simulink model "SAR_AOCS_Model"  (R2024a)
settings: Solver=VariableStepAuto  StartTime=0.0  StopTime=1000  RelTol=1e-3
values from neighbouring files (symbols this model uses):
  Q = 1e-10    [init_SAR_AOCS.m]
  Rgyro = 1e-12    [init_SAR_AOCS.m]
  Rstr = 1e-12    [init_SAR_AOCS.m]
  Ts = sim.dt    [init_SAR_AOCS.m]
  unit7 = ones(7,1)    [init_SAR_AOCS.m]
undefined symbols (not defined in the file or in its folder): initial, sim
libraries: simulink x3, slpidlib x3, sharedtransform x3, sharedTrackingLibrary x1, simulink_extras x1
settings Model: SimulationMode=accelerator  Creator=hendr  LastModifiedBy=hendr

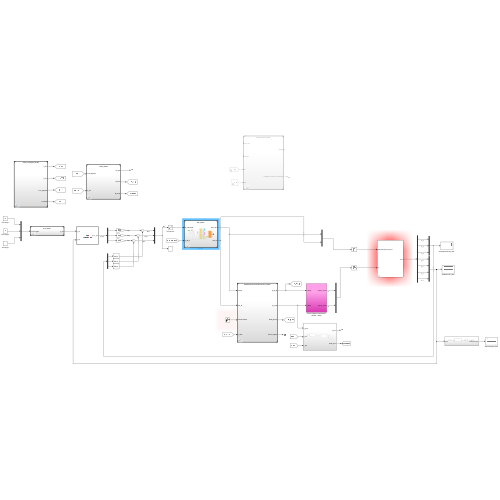
[thumbnail: Simulink's stored preview of the top-level diagram]
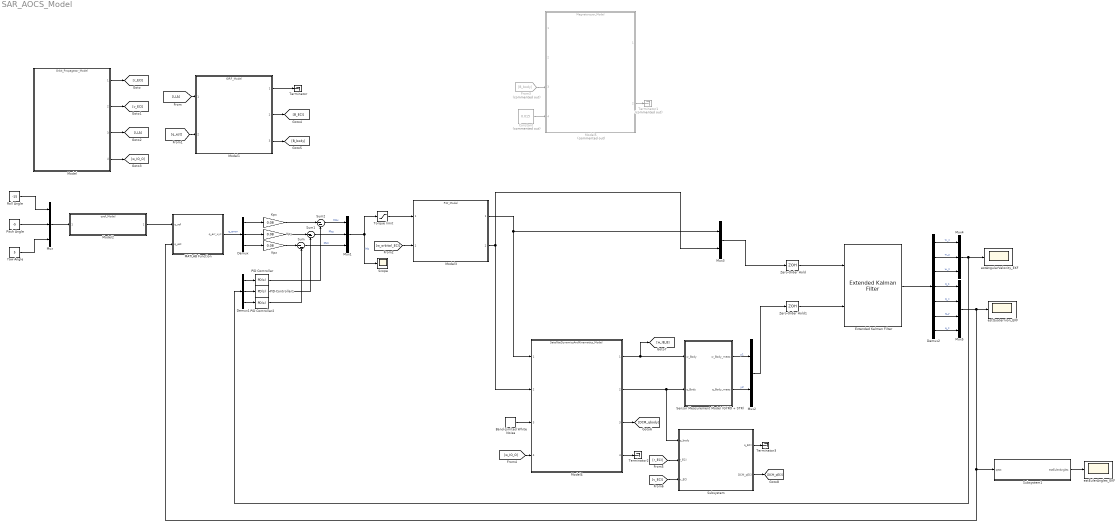
== system SAR_AOCS_Model ==
  Band-Limited White Noise : simulink/Sources/Band-Limited White Noise  Cov=Q*sim.dt  Ts=sim.dt  seed=[23341]
  Constant : Constant  Commented=on  Value=0.015
  Demux : Demux  Outputs=3
  Demux1 : Demux  Outputs=3
  Demux2 : Demux  Outputs=7
  Extended Kalman Filter : sharedTrackingLibrary/Extended Kalman Filter  StateTransitionFcn=dynamicFunctions2  HasStateTransitionJacobianFcn=off  HasAdditiveProcessNoise=Additive  ProcessNoise=diag(unit7)*Q  HasTimeVaryingProcessNoise=off  HasStateTransitionFcnExtraArgument=1  InitialState=[initial.omega, initial.q]  InitialStateCovariance=1e-6  MeasurementFcn1=measurementFunction2  HasMeasurementJacobianFcn1=off  HasMeasurementEnablePort1=off  HasAdditiveMeasurementNoise1=Additive  MeasurementNoise1=Rconf4  HasTimeVaryingMeasurementNoise1=off  HasMeasurementFcnExtraArgument1=0  HasMeasurementWrapping1=off  MeasurementFcn2=myMeasurementFcn  HasMeasurementJacobianFcn2=off  HasMeasurementEnablePort2=off  HasAdditiveMeasurementNoise2=Additive  MeasurementNoise2=1  HasTimeVaryingMeasurementNoise2=off  HasMeasurementFcnExtraArgument2=0  HasMeasurementWrapping2=off  MeasurementFcn3=myMeasurementFcn  HasMeasurementJacobianFcn3=off  HasMeasurementEnablePort3=off  HasAdditiveMeasurementNoise3=Additive  MeasurementNoise3=1  HasTimeVaryingMeasurementNoise3=off  HasMeasurementFcnExtraArgument3=0  HasMeasurementWrapping3=off  MeasurementFcn4=myMeasurementFcn  HasMeasurementJacobianFcn4=off  HasMeasurementEnablePort4=off  HasAdditiveMeasurementNoise4=Additive  MeasurementNoise4=1  HasTimeVaryingMeasurementNoise4=off  HasMeasurementFcnExtraArgument4=0  HasMeasurementWrapping4=off  MeasurementFcn5=myMeasurementFcn  HasMeasurementJacobianFcn5=off  HasMeasurementEnablePort5=off  HasAdditiveMeasurementNoise5=Additive  MeasurementNoise5=1  HasTimeVaryingMeasurementNoise5=off  HasMeasurementFcnExtraArgument5=0  HasMeasurementWrapping5=off  EnableMultirate=off  StateTransitionFcnSampleTime=1  MeasurementFcn1SampleTime=1  MeasurementFcn2SampleTime=1  MeasurementFcn3SampleTime=1  MeasurementFcn4SampleTime=1  MeasurementFcn5SampleTime=1  UseCurrentEstimator=on  OutputStateCovariance=off  DataType=double  SampleTime=Ts  NumberOfMeasurements=1
  From3 : From  Commented=on  GotoTag=B_body
  Kpx : Gain  Gain=0.08
  Kpy : Gain  Gain=0.08
  Kpz : Gain  Gain=0.08
  MATLAB Function : MATLAB Function  TreatAsAtomicUnit=on
  Model : ModelReference  ModelNameDialog=Orbit_Propagator_Model.slx  SimulationMode=Normal  ModelReferenceVersion=1.1
  Model1 : ModelReference  ModelNameDialog=IGRF_Model.slx  SimulationMode=Normal  ModelReferenceVersion=1.3
  Model2 : ModelReference  ModelNameDialog=qref_Model.slx  SimulationMode=Normal  ModelReferenceVersion=1.2
  Model3 : ModelReference  ModelNameDialog=RW_Model.slx  SimulationMode=Normal  ModelReferenceVersion=1.2
  Model4 : ModelReference  ModelNameDialog=SatelliteDynamicsAndKinematics_Model.slx  SimulationMode=Normal  ModelReferenceVersion=1.1
  Model5 : ModelReference  Commented=on  ModelNameDialog=Magnetorquer_Model.slx  SimulationMode=Normal  ModelReferenceVersion=1.3
  Mux : Mux  Inputs=3
  Mux1 : Mux  Inputs=3
  Mux2 : Mux  Inputs=2
  Mux3 : Mux  Inputs=2
  Mux4 : Mux  Inputs=3
  Mux5 : Mux
  PID Controller : slpidlib/PID Controller  Controller=PD  Form=Parallel  TimeDomain=Continuous-time  UseExternalTs=off  SampleTime=-1  IntegratorMethod=Forward Euler  FilterMethod=Forward Euler  ControllerParametersSource=internal  P=1  I=1  UseKiTs=off  D=2  UseExternalDerivativeSource=off  N=100  UseFilter=on  TunerSelectOption=Transfer Function Based (PID Tuner App)  InitialConditionSource=internal  InitialConditionForIntegrator=0  InitialConditionForFilter=0  DifferentiatorICPrevScaledInput=0  ExternalReset=none  TrackingMode=off  Kt=1  LimitOutput=off  SatLimitsSource=internal  UpperSaturationLimit=inf  LowerSaturationLimit=-inf  LinearizeAsGain=on  AntiWindupMode=none  Kb=1  LimitIntegrator=off  UpperIntegratorSaturationLimit=inf  LowerIntegratorSaturationLimit=-inf  POutMin=[]  POutMax=[]  IOutMin=[]  IOutMax=[]  DOutMin=[]  DOutMax=[]  NOutMin=[]  NOutMax=[]  SumOutMin=[]  SumOutMax=[]  SaturationOutMin=[]  SaturationOutMax=[]  PParamMin=[]  PParamMax=[]  IParamMin=[]  IParamMax=[]  DParamMin=[]  DParamMax=[]  NParamMin=[]  NParamMax=[]  KbParamMin=[]  KbParamMax=[]  KtParamMin=[]  KtParamMax=[]  KbOutMin=[]  KbOutMax=[]  KtOutMin=[]  KtOutMax=[]  IntegratorOutMin=[]  IntegratorOutMax=[]  FilterOutMin=[]  FilterOutMax=[]  SumI1OutMin=[]  SumI1OutMax=[]  SumI2OutMin=[]  SumI2OutMax=[]  SumI3OutMin=[]  SumI3OutMax=[]  SumI4OutMin=[]  SumI4OutMax=[]  SumDOutMin=[]  SumDOutMax=[]  DifferentiatorOutMin=[]  DifferentiatorOutMax=[]  FilterDiffOutCoefMin=[]  FilterDiffOutCoefMax=[]  ReciprocalOutMin=[]  ReciprocalOutMax=[]  SumDenOutMin=[]  SumDenOutMax=[]  SumNumOutMin=[]  SumNumOutMax=[]  DivideOutMin=[]  DivideOutMax=[]  UdiffTsProdOutMin=[]  UdiffTsProdOutMax=[]  NTsProdOutMin=[]  NTsProdOutMax=[]  UintegralTsProdOutMin=[]  UintegralTsProdOutMax=[]  UngainTsProdOutMin=[]  UngainTsProdOutMax=[]  ClampingZeroOutDataTypeStr=Inherit: Inherit via back propagation  ClampingZeroOutMin=[]  ClampingZeroOutMax=[]  FilterDenConstantOutDataTypeStr=Inherit: Inherit via back propagation  FilterDenConstantOutMin=[]  FilterDenConstantOutMax=[]  PCopyOutDataTypeStr=Inherit: Inherit via back propagation  PCopyOutMin=[]  PCopyOutMax=[]  NCopyOutDataTypeStr=Inherit: Inherit via back propagation  NCopyOutMin=[]  NCopyOutMax=[]  IntegratorContinuousStateAttributes=''  IntegratorStateMustResolveToSignalObject=off  IntegratorRTWStateStorageClass=Auto  FilterContinuousStateAttributes=''  FilterStateMustResolveToSignalObject=off  FilterRTWStateStorageClass=Auto  ParallelPVariant=InternalParameters  IdealPVariant=Disabled  IVariant=Disabled  DVariant=InternalParameters  IntegratorVariant=Disabled  SatVariant=Disabled  AWVariant=Disabled  PCopyVariant=Disabled  TRVariant=Disabled  FdbkBlocksVariant=Forward  IdealPFdbkVariant=Disabled  SatFdbkVariant=Disabled  DerivativeFilterVariant=ContFilter  NVariant=InternalParameters  NCopyVariant=Disabled  FilterICVariant=InternalICsFilter  IntegratorICVariant=Disabled  ExternalResetVariant=Disabled  TRSumVariant=Passthrough  SumFdbkVariant=Disabled  SumVariant=Sum_PD  TsampFilterVariant=InternalTs  TsampNgainVariant=Passthrough  TsampIntegralVariant=Disabled_SignalSpec  ExternalSaturationOutDataTypeStr=Inherit: Same as second input  DerivativeSourceVariant=ErrorSignal
  PID Controller1 : slpidlib/PID Controller  Controller=PD  Form=Parallel  TimeDomain=Continuous-time  UseExternalTs=off  SampleTime=-1  IntegratorMethod=Forward Euler  FilterMethod=Forward Euler  ControllerParametersSource=internal  P=1  I=1  UseKiTs=off  D=2  UseExternalDerivativeSource=off  N=100  UseFilter=on  TunerSelectOption=Transfer Function Based (PID Tuner App)  InitialConditionSource=internal  InitialConditionForIntegrator=0  InitialConditionForFilter=0  DifferentiatorICPrevScaledInput=0  ExternalReset=none  TrackingMode=off  Kt=1  LimitOutput=off  SatLimitsSource=internal  UpperSaturationLimit=inf  LowerSaturationLimit=-inf  LinearizeAsGain=on  AntiWindupMode=none  Kb=1  LimitIntegrator=off  UpperIntegratorSaturationLimit=inf  LowerIntegratorSaturationLimit=-inf  POutMin=[]  POutMax=[]  IOutMin=[]  IOutMax=[]  DOutMin=[]  DOutMax=[]  NOutMin=[]  NOutMax=[]  SumOutMin=[]  SumOutMax=[]  SaturationOutMin=[]  SaturationOutMax=[]  PParamMin=[]  PParamMax=[]  IParamMin=[]  IParamMax=[]  DParamMin=[]  DParamMax=[]  NParamMin=[]  NParamMax=[]  KbParamMin=[]  KbParamMax=[]  KtParamMin=[]  KtParamMax=[]  KbOutMin=[]  KbOutMax=[]  KtOutMin=[]  KtOutMax=[]  IntegratorOutMin=[]  IntegratorOutMax=[]  FilterOutMin=[]  FilterOutMax=[]  SumI1OutMin=[]  SumI1OutMax=[]  SumI2OutMin=[]  SumI2OutMax=[]  SumI3OutMin=[]  SumI3OutMax=[]  SumI4OutMin=[]  SumI4OutMax=[]  SumDOutMin=[]  SumDOutMax=[]  DifferentiatorOutMin=[]  DifferentiatorOutMax=[]  FilterDiffOutCoefMin=[]  FilterDiffOutCoefMax=[]  ReciprocalOutMin=[]  ReciprocalOutMax=[]  SumDenOutMin=[]  SumDenOutMax=[]  SumNumOutMin=[]  SumNumOutMax=[]  DivideOutMin=[]  DivideOutMax=[]  UdiffTsProdOutMin=[]  UdiffTsProdOutMax=[]  NTsProdOutMin=[]  NTsProdOutMax=[]  UintegralTsProdOutMin=[]  UintegralTsProdOutMax=[]  UngainTsProdOutMin=[]  UngainTsProdOutMax=[]  ClampingZeroOutDataTypeStr=Inherit: Inherit via back propagation  ClampingZeroOutMin=[]  ClampingZeroOutMax=[]  FilterDenConstantOutDataTypeStr=Inherit: Inherit via back propagation  FilterDenConstantOutMin=[]  FilterDenConstantOutMax=[]  PCopyOutDataTypeStr=Inherit: Inherit via back propagation  PCopyOutMin=[]  PCopyOutMax=[]  NCopyOutDataTypeStr=Inherit: Inherit via back propagation  NCopyOutMin=[]  NCopyOutMax=[]  IntegratorContinuousStateAttributes=''  IntegratorStateMustResolveToSignalObject=off  IntegratorRTWStateStorageClass=Auto  FilterContinuousStateAttributes=''  FilterStateMustResolveToSignalObject=off  FilterRTWStateStorageClass=Auto  ParallelPVariant=InternalParameters  IdealPVariant=Disabled  IVariant=Disabled  DVariant=InternalParameters  IntegratorVariant=Disabled  SatVariant=Disabled  AWVariant=Disabled  PCopyVariant=Disabled  TRVariant=Disabled  FdbkBlocksVariant=Forward  IdealPFdbkVariant=Disabled  SatFdbkVariant=Disabled  DerivativeFilterVariant=ContFilter  NVariant=InternalParameters  NCopyVariant=Disabled  FilterICVariant=InternalICsFilter  IntegratorICVariant=Disabled  ExternalResetVariant=Disabled  TRSumVariant=Passthrough  SumFdbkVariant=Disabled  SumVariant=Sum_PD  TsampFilterVariant=InternalTs  TsampNgainVariant=Passthrough  TsampIntegralVariant=Disabled_SignalSpec  ExternalSaturationOutDataTypeStr=Inherit: Same as second input  DerivativeSourceVariant=ErrorSignal
  PID Controller2 : slpidlib/PID Controller  Controller=PD  Form=Parallel  TimeDomain=Continuous-time  UseExternalTs=off  SampleTime=-1  IntegratorMethod=Forward Euler  FilterMethod=Forward Euler  ControllerParametersSource=internal  P=1  I=1  UseKiTs=off  D=2  UseExternalDerivativeSource=off  N=100  UseFilter=on  TunerSelectOption=Transfer Function Based (PID Tuner App)  InitialConditionSource=internal  InitialConditionForIntegrator=0  InitialConditionForFilter=0  DifferentiatorICPrevScaledInput=0  ExternalReset=none  TrackingMode=off  Kt=1  LimitOutput=off  SatLimitsSource=internal  UpperSaturationLimit=inf  LowerSaturationLimit=-inf  LinearizeAsGain=on  AntiWindupMode=none  Kb=1  LimitIntegrator=off  UpperIntegratorSaturationLimit=inf  LowerIntegratorSaturationLimit=-inf  POutMin=[]  POutMax=[]  IOutMin=[]  IOutMax=[]  DOutMin=[]  DOutMax=[]  NOutMin=[]  NOutMax=[]  SumOutMin=[]  SumOutMax=[]  SaturationOutMin=[]  SaturationOutMax=[]  PParamMin=[]  PParamMax=[]  IParamMin=[]  IParamMax=[]  DParamMin=[]  DParamMax=[]  NParamMin=[]  NParamMax=[]  KbParamMin=[]  KbParamMax=[]  KtParamMin=[]  KtParamMax=[]  KbOutMin=[]  KbOutMax=[]  KtOutMin=[]  KtOutMax=[]  IntegratorOutMin=[]  IntegratorOutMax=[]  FilterOutMin=[]  FilterOutMax=[]  SumI1OutMin=[]  SumI1OutMax=[]  SumI2OutMin=[]  SumI2OutMax=[]  SumI3OutMin=[]  SumI3OutMax=[]  SumI4OutMin=[]  SumI4OutMax=[]  SumDOutMin=[]  SumDOutMax=[]  DifferentiatorOutMin=[]  DifferentiatorOutMax=[]  FilterDiffOutCoefMin=[]  FilterDiffOutCoefMax=[]  ReciprocalOutMin=[]  ReciprocalOutMax=[]  SumDenOutMin=[]  SumDenOutMax=[]  SumNumOutMin=[]  SumNumOutMax=[]  DivideOutMin=[]  DivideOutMax=[]  UdiffTsProdOutMin=[]  UdiffTsProdOutMax=[]  NTsProdOutMin=[]  NTsProdOutMax=[]  UintegralTsProdOutMin=[]  UintegralTsProdOutMax=[]  UngainTsProdOutMin=[]  UngainTsProdOutMax=[]  ClampingZeroOutDataTypeStr=Inherit: Inherit via back propagation  ClampingZeroOutMin=[]  ClampingZeroOutMax=[]  FilterDenConstantOutDataTypeStr=Inherit: Inherit via back propagation  FilterDenConstantOutMin=[]  FilterDenConstantOutMax=[]  PCopyOutDataTypeStr=Inherit: Inherit via back propagation  PCopyOutMin=[]  PCopyOutMax=[]  NCopyOutDataTypeStr=Inherit: Inherit via back propagation  NCopyOutMin=[]  NCopyOutMax=[]  IntegratorContinuousStateAttributes=''  IntegratorStateMustResolveToSignalObject=off  IntegratorRTWStateStorageClass=Auto  FilterContinuousStateAttributes=''  FilterStateMustResolveToSignalObject=off  FilterRTWStateStorageClass=Auto  ParallelPVariant=InternalParameters  IdealPVariant=Disabled  IVariant=Disabled  DVariant=InternalParameters  IntegratorVariant=Disabled  SatVariant=Disabled  AWVariant=Disabled  PCopyVariant=Disabled  TRVariant=Disabled  FdbkBlocksVariant=Forward  IdealPFdbkVariant=Disabled  SatFdbkVariant=Disabled  DerivativeFilterVariant=ContFilter  NVariant=InternalParameters  NCopyVariant=Disabled  FilterICVariant=InternalICsFilter  IntegratorICVariant=Disabled  ExternalResetVariant=Disabled  TRSumVariant=Passthrough  SumFdbkVariant=Disabled  SumVariant=Sum_PD  TsampFilterVariant=InternalTs  TsampNgainVariant=Passthrough  TsampIntegralVariant=Disabled_SignalSpec  ExternalSaturationOutDataTypeStr=Inherit: Same as second input  DerivativeSourceVariant=ErrorSignal
  Pitch Angle : Constant  Value=-5
  Roll Angle : Constant  Value=-15
  Scope : Scope
  Sensor Measurement Model (GYRO + STR) : Subsystem
  Subsystem : Subsystem
  Subsystem1 : Subsystem
  Sum : Sum  Inputs=|--
  Sum1 : Sum  Inputs=|--
  Sum2 : Sum  Inputs=|--
  Terminator : Terminator
  Terminator1 : Terminator  Commented=on
  Terminator2 : Terminator
  Terminator3 : Terminator
  Torque limit : Saturate
  Yaw Angle : Constant  Value=5
  Zero-Order Hold : ZeroOrderHold  SampleTime=sim.dt
  Zero-Order Hold1 : ZeroOrderHold  SampleTime=sim.dt
  estAngularVelocity_EKF : Scope
  estEulerAngles_EKF : Scope
  estQuaternion_EKF : Scope
  wires:
  Model/1 -> [r_ECI]
  Model/2 -> [v_ECI]
  Model/3 -> [LLA]
  Model/4 -> [w_IO_O]
  [LLA] -> Model1/1
  Model1/2 -> [B_ECI]
  Roll Angle/1 -> Mux/1
  Pitch Angle/1 -> Mux/2
  Yaw Angle/1 -> Mux/3
  Mux/1 -> Model2/1
  Model2/1 -> MATLAB Function/1(q_ref)
  MATLAB Function/1(q_err_xyz) -> Demux/1  "q_error"
  Demux/3 -> Kpz/1
  Demux/2 -> Kpy/1
  Demux/1 -> Kpx/1
  Kpz/1 -> Sum/1
  Kpx/1 -> Sum2/1
  Kpy/1 -> Sum1/1
  Sum2/1 -> Mux1/1  "Mcx"
  Sum1/1 -> Mux1/2  "Mcy"
  Sum/1 -> Mux1/3  "Mcz"
  Demux1/1 -> PID Controller/1
  PID Controller/1 -> Sum2/2
  Demux1/2 -> PID Controller1/1
  Demux1/3 -> PID Controller2/1
  PID Controller1/1 -> Sum1/2
  PID Controller2/1 -> Sum/2
  [q_est] -> Model1/2
  Model1/3 -> [B_body]
  Model1/1 -> Terminator/1
  Mux1/1 -> Scope/1, Torque limit/1  "Mc"
  [w_orbital_ECI] -> Model3/2
  Torque limit/1 -> Model3/1
  Model3/2 -> Model4/2, Mux3/2
  From3/1 -> Model5/3
  Constant/1 -> Model5/4
  Band-Limited White Noise/1 -> Model4/3
  [w_IO_O] -> Model4/4
  Model4/3 -> [DCM_qbody]
  Model4/1 -> Sensor Measurement Model (GYRO + STR)/1(w_Body), [w_IB_B]
  Model5/2 -> Terminator1/1
  Model4/2 -> Subsystem/1(q_body), Sensor Measurement Model (GYRO + STR)/2(q_Body)
  Sensor Measurement Model (GYRO + STR)/1(w_Body_meas) -> Mux2/1  "y1"
  Sensor Measurement Model (GYRO + STR)/2(q_Body_meas) -> Mux2/2  "y2"
  Model4/4 -> Terminator2/1
  [r_ECI] -> Subsystem/2(r_ECI)
  [v_ECI] -> Subsystem/3(v_ECI)
  Subsystem/1(q_ECI) -> Terminator3/1
  Subsystem/2(DCM_qECI) -> [DCM_qECI]
  Mux3/1 -> Zero-Order Hold/1
  Mux2/1 -> Zero-Order Hold1/1
  Zero-Order Hold/1 -> Extended Kalman Filter/1
  Zero-Order Hold1/1 -> Extended Kalman Filter/2
  Extended Kalman Filter/1 -> Demux2/1
  Demux2/1 -> Mux4/1  "w_x"
  Demux2/2 -> Mux4/2  "w_y"
  Demux2/3 -> Mux4/3  "w_z"
  Demux2/5 -> Mux5/2  "q_x"
  Demux2/6 -> Mux5/3  "q_y"
  Demux2/7 -> Mux5/4  "q_z"
  Demux2/4 -> Mux5/1  "q_s"
  Mux4/1 -> estAngularVelocity_EKF/1, Demux1/1
  Mux5/1 -> estQuaternion_EKF/1, Subsystem1/1(qest), MATLAB Function/2(q_est)
  Subsystem1/1(estEulerAngles) -> estEulerAngles_EKF/1
  Model3/1 -> Mux3/1, Model4/1

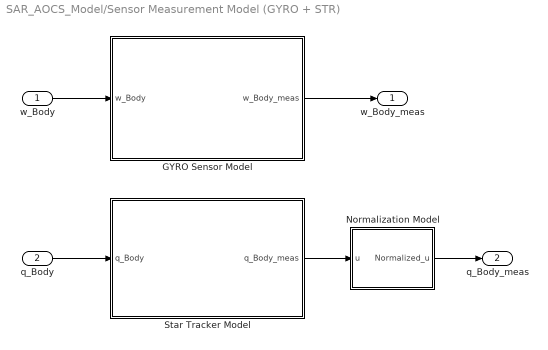
== system SAR_AOCS_Model/Sensor Measurement Model (GYRO + STR) ==
  w_Body : Inport
  q_Body : Inport  Port=2
  GYRO Sensor Model : Subsystem
  Normalization Model : Subsystem
  Star Tracker Model : Subsystem
  w_Body_meas : Outport  VectorParamsAs1DForOutWhenUnconnected=off
  q_Body_meas : Outport  Port=2  VectorParamsAs1DForOutWhenUnconnected=off
  wires:
  GYRO Sensor Model/1(w_Body_meas) -> w_Body_meas/1
  w_Body/1 -> GYRO Sensor Model/1(w_Body)
  q_Body/1 -> Star Tracker Model/1(q_Body)
  Normalization Model/1(Normalized_u) -> q_Body_meas/1
  Star Tracker Model/1(q_Body_meas) -> Normalization Model/1(u)

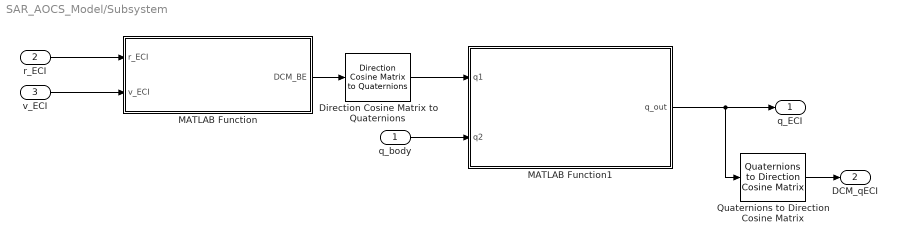
== system SAR_AOCS_Model/Subsystem ==
  q_body : Inport
  r_ECI : Inport  Port=2
  v_ECI : Inport  Port=3
  Direction Cosine Matrix to Quaternions : sharedtransform/Direction Cosine Matrix  to Quaternions  aMode=0  action=None  tolerance=eps(2)
      settings: LibrarySourceBlock=|
      | aerolibtransform2/Direction Cosine Matrix
      | to Quaternions
  MATLAB Function : MATLAB Function  TreatAsAtomicUnit=on
  MATLAB Function1 : MATLAB Function  TreatAsAtomicUnit=on
  Quaternions to Direction Cosine Matrix : sharedtransform/Quaternions to  Direction Cosine Matrix  aMode=aMode
      settings: LibrarySourceBlock=|
      | aerolibtransform2/Quaternions to
      | Direction Cosine Matrix
  q_ECI : Outport
  DCM_qECI : Outport  Port=2
  wires:
  MATLAB Function/1(DCM_BE) -> Direction Cosine Matrix to Quaternions/1
  r_ECI/1 -> MATLAB Function/1(r_ECI)
  v_ECI/1 -> MATLAB Function/2(v_ECI)
  q_body/1 -> MATLAB Function1/2(q2)
  Direction Cosine Matrix to Quaternions/1 -> MATLAB Function1/1(q1)
  MATLAB Function1/1(q_out) -> Quaternions to Direction Cosine Matrix/1, q_ECI/1
  Quaternions to Direction Cosine Matrix/1 -> DCM_qECI/1

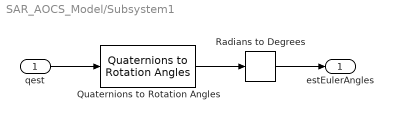
== system SAR_AOCS_Model/Subsystem1 ==
  qest : Inport
  Quaternions to Rotation Angles : sharedtransform/Quaternions to Rotation Angles  rotationOrder=ZYX  aMode=aMode
  Radians to Degrees : simulink_extras/Transformations/Radians to Degrees
  estEulerAngles : Outport
  wires:
  qest/1 -> Quaternions to Rotation Angles/1
  Quaternions to Rotation Angles/1 -> Radians to Degrees/1
  Radians to Degrees/1 -> estEulerAngles/1

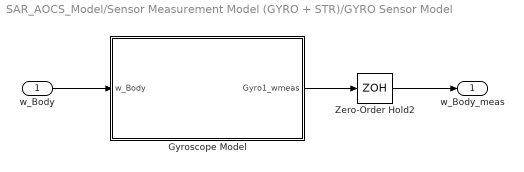
== system SAR_AOCS_Model/Sensor Measurement Model (GYRO + STR)/GYRO Sensor Model ==
  w_Body : Inport
  Gyroscope Model : Subsystem
  Zero-Order Hold2 : ZeroOrderHold  SampleTime=Ts
  w_Body_meas : Outport  VectorParamsAs1DForOutWhenUnconnected=off
  wires:
  w_Body/1 -> Gyroscope Model/1(w_Body)
  Gyroscope Model/1(Gyro1_wmeas) -> Zero-Order Hold2/1
  Zero-Order Hold2/1 -> w_Body_meas/1

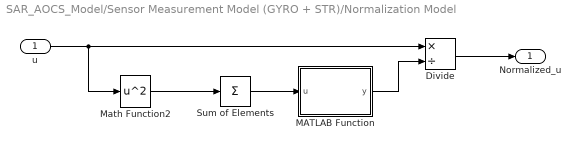
== system SAR_AOCS_Model/Sensor Measurement Model (GYRO + STR)/Normalization Model ==
  u : Inport
  Divide : Product  Inputs=*/
  MATLAB Function : MATLAB Function  TreatAsAtomicUnit=on
  Math Function2 : Math  Operator=square  SignedPower=on
  Sum of Elements : Sum  Inputs=+
  Normalized_u : Outport  VectorParamsAs1DForOutWhenUnconnected=off
  wires:
  Divide/1 -> Normalized_u/1
  MATLAB Function/1(y) -> Divide/2
  Sum of Elements/1 -> MATLAB Function/1(u)
  u/1 -> Divide/1, Math Function2/1
  Math Function2/1 -> Sum of Elements/1

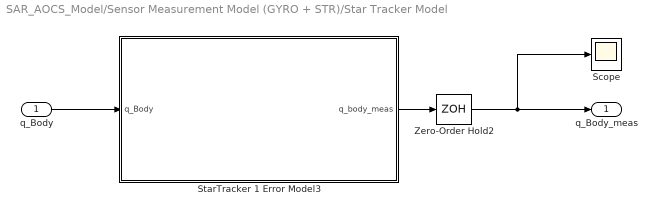
== system SAR_AOCS_Model/Sensor Measurement Model (GYRO + STR)/Star Tracker Model ==
  q_Body : Inport
  Scope : Scope
  StarTracker 1 Error Model3 : Subsystem  TreatAsAtomicUnit=on
  Zero-Order Hold2 : ZeroOrderHold  SampleTime=0.1
  q_Body_meas : Outport  VectorParamsAs1DForOutWhenUnconnected=off
  wires:
  Zero-Order Hold2/1 -> Scope/1, q_Body_meas/1
  q_Body/1 -> StarTracker 1 Error Model3/1("q_Body ")
  StarTracker 1 Error Model3/1("q_body_meas ") -> Zero-Order Hold2/1

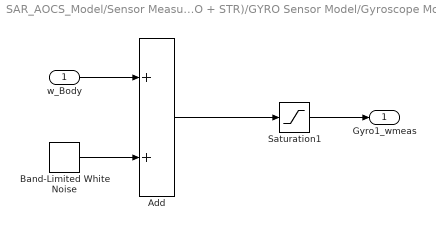
== system SAR_AOCS_Model/Sensor Measurement Model (GYRO + STR)/GYRO Sensor Model/Gyroscope Model ==
  w_Body : Inport
  Add : Sum
  Band-Limited White Noise : simulink/Sources/Band-Limited White Noise  Cov=Rgyro*Ts  Ts=Ts  seed=[23341]
  Saturation1 : Saturate  UpperLimit=abs(1000)  LowerLimit=-abs(1000)
  Gyro1_wmeas : Outport  VectorParamsAs1DForOutWhenUnconnected=off
  wires:
  Add/1 -> Saturation1/1
  Saturation1/1 -> Gyro1_wmeas/1
  w_Body/1 -> Add/1
  Band-Limited White Noise/1 -> Add/2

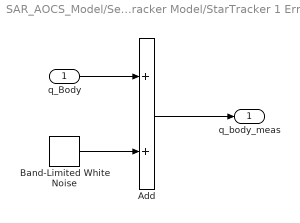
== system SAR_AOCS_Model/Sensor Measurement Model (GYRO + STR)/Star Tracker Model/StarTracker 1 Error Model3 ==
  "q_Body " : Inport
  Add : Sum
  Band-Limited White Noise : simulink/Sources/Band-Limited White Noise  Cov=Rstr*Ts  Ts=Ts  seed=[12345]
  "q_body_meas " : Outport  VectorParamsAs1DForOutWhenUnconnected=off
  wires:
  Band-Limited White Noise/1 -> Add/2
  "q_Body "/1 -> Add/1
  Add/1 -> "q_body_meas "/1

== matlab function SAR_AOCS_Model/MATLAB Function ==
  data: q_ref input; q_est input; q_err_xyz output
function q_err_xyz  = quaternion_error(q_ref, q_est)
% QUATERNION_ERROR
% Computes the multiplicative quaternion error
%
% Inputs:
%   q_est : 4x1 estimated quaternion [w; x; y; z]
%   q_ref : 4x1 reference quaternion [w; x; y; z]
%
% Output:
%   q_err : 4x1 error quaternion [w; x; y; z]
%   q_err_xyz : 3x1 error quaternion [x; y; z]


% Ensure column vectors
q_est = q_est(:);
q_ref = q_ref(:);

% Ensure Normalized for numerical stability
q_ref = q_ref / norm(q_ref);
q_est = q_est / norm(q_est);

% Compute error quaternion: δq = q_est ⊗ q_ref^(-1)
q_ref_inv = [q_ref(1); -q_ref(2:4)]; % conjugate = inverse for unit quat
q_err = quat_multiply(q_est, q_ref_inv);
q_err_xyz = q_err(2:4);

end


function q_out = quat_multiply(q1, q2)
w1 = q1(1);
x1 = q1(2);
y1 = q1(3);
z1 = q1(4);

w2 = q2(1);
x2 = q2(2);
y2 = q2(3);
z2 = q2(4);

q_out = [(w1*w2 - x1*x2 - y1*y2 - z1*z2)
    (w1*x2 + x1*w2 + y1*z2 - z1*y2)
    (w1*y2 - x1*z2 + y1*w2 + z1*x2)
    (w1*z2 + x1*y2 - y1*x2 + z1*w2)];

end

== matlab function SAR_AOCS_Model/Subsystem/MATLAB Function1 ==
  data: q1 input; q_out output; q2 input
function q_out = quat_multiply(q1, q2)
w1 = q1(1);
x1 = q1(2);
y1 = q1(3);
z1 = q1(4);

w2 = q2(1);
x2 = q2(2);
y2 = q2(3);
z2 = q2(4);

q_out = [(w1*w2 - x1*x2 - y1*y2 - z1*z2)
    (w1*x2 + x1*w2 + y1*z2 - z1*y2)
    (w1*y2 - x1*z2 + y1*w2 + z1*x2)
    (w1*z2 + x1*y2 - y1*x2 + z1*w2)];

end

== matlab function SAR_AOCS_Model/Sensor Measurement Model (GYRO + STR)/Normalization Model/MATLAB Function ==
  data: u input; y output
function y = Sqrt(u)
%#codegen

y = sqrt(u);

== matlab function SAR_AOCS_Model/Subsystem/MATLAB Function ==
  data: r_ECI input; DCM_BE output; v_ECI input
function DCM_BE = ECI_to_LVLH(r_ECI, v_ECI)

%--------------------------------------------------------------------------
% Converts ECI position/velocity vectors into LVLH DCM
%
% Inputs:
%   r_ECI  [3x1] position vector in ECI frame (m)
%   v_ECI  [3x1] velocity vector in ECI frame (m/s)
%
% Output:
%   DCM_LE [3x3] Direction Cosine Matrix:
%                ECI --> LVLH
%
% LVLH Convention:
%   x-axis : radial outward
%   y-axis : along-track
%   z-axis : orbit normal
%
% Right-handed frame
%--------------------------------------------------------------------------

% Normalize radial direction

x_hat = r_ECI / norm(r_ECI);

% Orbit angular momentum vector

h = cross(r_ECI, v_ECI);

% Orbit normal direction

z_hat = h / norm(h);

% Along-track direction

y_hat = cross(z_hat, x_hat);

% Normalize for numerical robustness

y_hat = y_hat / norm(y_hat);

% Construct LVLH-to-ECI DCM

DCM_EL = [x_hat, y_hat, z_hat];

% Convert ECI -> LVLH

DCM_LE = DCM_EL';

% Assuming the spacecraft body frame is aligned with LVLH

DCM_BE = DCM_LE;

end
